simulink library "isi_correlator_lib"  (Simulink 7.3)
settings: Solver=ode45  SolverMode=SingleTasking  StartTime=0.0  StopTime=10.0  RelTol=1e-3
libraries: xbsIndex_r4 x337, casper_library x37, xps_library x31, isi_correlator_lib x28
(part 3 of 3)

== system isi_correlator_lib/capt_xaui/capt1 ==
  din0 : Inport
  din1 : Inport  Port=2
  din2 : Inport  Port=3
  en : Inport  Port=4
  trig : Inport  Port=5
  Constant : xbsIndex_r4/Constant  arith_type=Boolean  const=1  n_bits=1  bin_pt=0  explicit_period=on  period=1  equ=P=C  opselect=C  inp2=PCIN>>17  opr=+  inp1=P  carry=CIN  dbl_ovrd=off  block_type=constant
      settings: block_version=11.3
  Logical : xbsIndex_r4/Logical  logical_function=AND  inputs=2  en=off  latency=0  precision=Full  arith_type=Unsigned  n_bits=16  bin_pt=0  align_bp=on  dbl_ovrd=off  block_type=logical
      settings: block_version=11.3
  bram0 : xps_library/Shared BRAM  Tag=xps:bram  SystemSampleTime=-1  arith_type=Unsigned  addr_width=addr_width  data_width=32  data_bin_pt=0  init_vals=0  sample_rate=1
  bram1 : xps_library/Shared BRAM  Tag=xps:bram  SystemSampleTime=-1  arith_type=Unsigned  addr_width=addr_width  data_width=32  data_bin_pt=0  init_vals=0  sample_rate=1
  bram2 : xps_library/Shared BRAM  Tag=xps:bram  SystemSampleTime=-1  arith_type=Unsigned  addr_width=addr_width  data_width=32  data_bin_pt=0  init_vals=0  sample_rate=1
  freeze_cntr : casper_library/Misc/freeze_cntr  SystemSampleTime=-1  CounterBits=addr_width
  reinterp0 : xbsIndex_r4/Reinterpret  force_arith_type=on  arith_type=Unsigned  force_bin_pt=on  bin_pt=0  block_type=reinterpret
      settings: infoedit="Changes signal type without altering the binary representation.   You can changed the signal between signed and unsigned, and relocate the binary point.<br><br>Hardware notes: In hardware this block costs nothing.<br><br>Example:  Suppose the input is 6 bits wide, signed, with 2 fractional bits, and the output is forced to unsigned with 0 fractional bits.  Then an input of -2.0 (1110.00 in binary 2's complement) becomes an output of 56 (111000 in binary)."  block_version=11.3
  reinterp1 : xbsIndex_r4/Reinterpret  force_arith_type=on  arith_type=Unsigned  force_bin_pt=on  bin_pt=0  block_type=reinterpret
      settings: infoedit="Changes signal type without altering the binary representation.   You can changed the signal between signed and unsigned, and relocate the binary point.<br><br>Hardware notes: In hardware this block costs nothing.<br><br>Example:  Suppose the input is 6 bits wide, signed, with 2 fractional bits, and the output is forced to unsigned with 0 fractional bits.  Then an input of -2.0 (1110.00 in binary 2's complement) becomes an output of 56 (111000 in binary)."  block_version=11.3
  reinterp2 : xbsIndex_r4/Reinterpret  force_arith_type=on  arith_type=Unsigned  force_bin_pt=on  bin_pt=0  block_type=reinterpret
      settings: infoedit="Changes signal type without altering the binary representation.   You can changed the signal between signed and unsigned, and relocate the binary point.<br><br>Hardware notes: In hardware this block costs nothing.<br><br>Example:  Suppose the input is 6 bits wide, signed, with 2 fractional bits, and the output is forced to unsigned with 0 fractional bits.  Then an input of -2.0 (1110.00 in binary 2's complement) becomes an output of 56 (111000 in binary)."  block_version=11.3
  terminator0 : Terminator
  terminator1 : Terminator
  terminator2 : Terminator
  terminator_done : Terminator
  wires:
  din0/1 -> reinterp0/1
  reinterp0/1 -> bram0/2
  bram0/1 -> terminator0/1
  din1/1 -> reinterp1/1
  reinterp1/1 -> bram1/2
  bram1/1 -> terminator1/1
  din2/1 -> reinterp2/1
  reinterp2/1 -> bram2/2
  bram2/1 -> terminator2/1
  freeze_cntr/3 -> terminator_done/1
  en/1 -> Logical/1
  trig/1 -> Logical/2
  Constant/1 -> freeze_cntr/1
  Logical/1 -> freeze_cntr/2
  freeze_cntr/1 -> bram0/1, bram1/1, bram2/1
  freeze_cntr/2 -> bram0/3, bram1/3, bram2/3
